simulink library "customLookUpTable"  (R2016b)
settings: Solver=VariableStepAuto  StartTime=0.0  StopTime=10.0  RelTol=1e-3
settings Model: Creator=lucadelaat  LastModifiedBy=lucadelaat

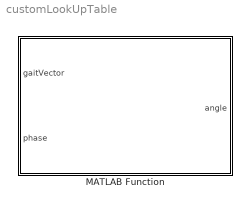
== system customLookUpTable ==
  MATLAB Function : MATLAB Function  TreatAsAtomicUnit=on

== matlab function customLookUpTable/MATLAB Function ==
  data: gaitVector input; angle output; phase input
function angle  = lookup_table(gaitVector, phase)
% wrapper for lookup_table
[angle] = lookup_table(gaitVector, phase);
end
